simulink model "sampleModel2001_1_sub_sub_sub"  (R2023a)
settings: Solver=VariableStepAuto  StartTime=0.0  StopTime=10.0  RelTol=1e-3
libraries: hdlsllib x4, simulink x1
settings Model: Creator=user1  LastModifiedBy=user1
settings OptimizationCC: BlockReduction=off  ConditionallyExecuteInputs=off

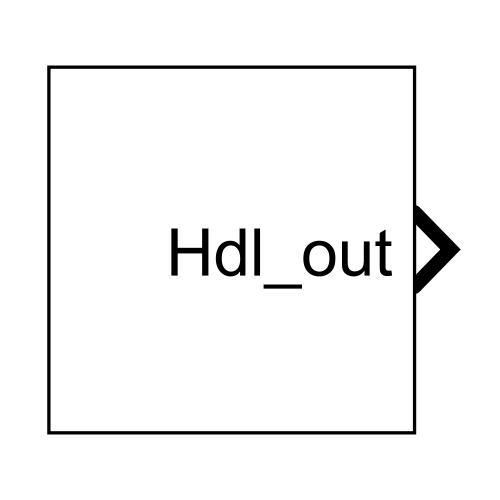
[thumbnail: Simulink's stored preview of the top-level diagram]
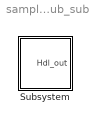
== system sampleModel2001_1_sub_sub_sub ==
  Subsystem : Subsystem

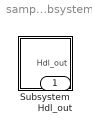
== system sampleModel2001_1_sub_sub_sub/Subsystem ==
  Subsystem : Subsystem
  Hdl_out : Outport  OutDataTypeStr=uint8

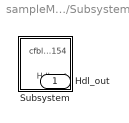
== system sampleModel2001_1_sub_sub_sub/Subsystem/Subsystem ==
  Subsystem : Subsystem
  Hdl_out : Outport  OutDataTypeStr=uint8

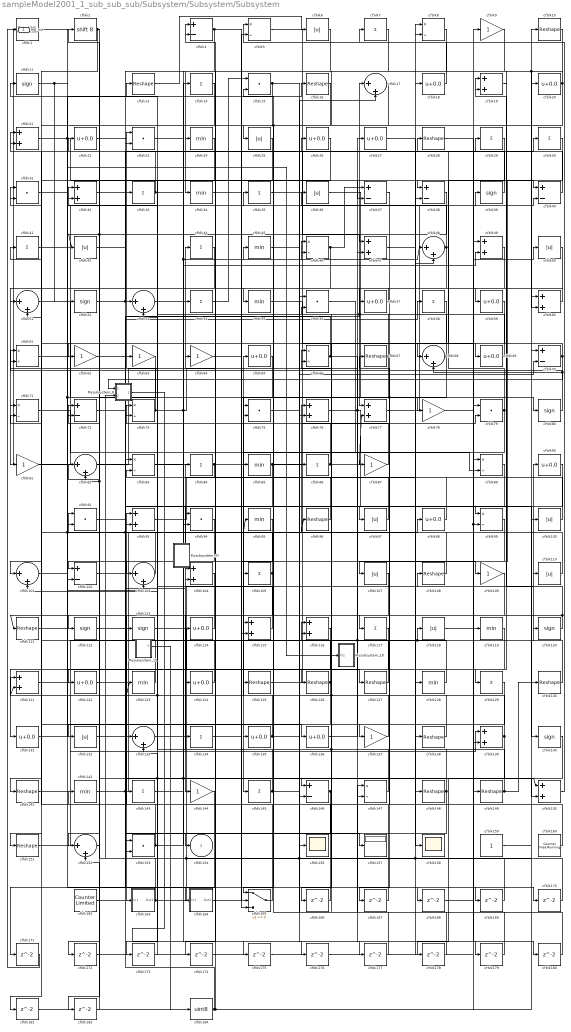
== system sampleModel2001_1_sub_sub_sub/Subsystem/Subsystem/Subsystem ==
  Mysubsystem_11 : Subsystem  TreatAsAtomicUnit=on  RTWFcnName=Mysubsystem_11
      settings: RTWFcnNameOpts=User specified  RTWFileNameOpts=Use function name
  Mysubsystem_19 : Subsystem  TreatAsAtomicUnit=on  RTWFcnName=Mysubsystem_19
      settings: RTWFcnNameOpts=User specified  RTWFileNameOpts=Use function name
  Mysubsystem_37 : Subsystem  TreatAsAtomicUnit=on  RTWFcnName=Mysubsystem_37
      settings: RTWFcnNameOpts=User specified  RTWFileNameOpts=Use function name
  Mysubsystem_8 : Subsystem  TreatAsAtomicUnit=on  RTWFcnName=Mysubsystem_8
      settings: RTWFcnNameOpts=User specified  RTWFileNameOpts=Use function name
  cfblk1 : hdlsllib/Logic and Bit Operations/Detect Fall Nonpositive  vinit=0  OutDataTypeStr=uint8
  cfblk{10,13,16,28,67,96,108,111,125..127,130,138,141,148..149,151} (17 alike) : Reshape
  cfblk{6,25,36,42,50,97,100,107,110,118,132} (11 alike) : Abs  OutDataTypeStr=uint8  SaturateOnIntegerOverflow=off
  cfblk{17,48,51,53,68,82,101,103,133,152} (10 alike) : Sum  Inputs=|++  OutDataTypeStr=uint8
  cfblk{4,37..38,40,70,72,102,146} (8 alike) : Sum  Inputs=+-  OutDataTypeStr=uint8
  cfblk{19,21,32,47,49,60,76..77,93,104,115..116,121,139,150} (15 alike) : Sum  OutDataTypeStr=uint8
  cfblk{7,14,29..30,33,35,41,44,54,58,84,86,105,117,129,134,143,145} (18 alike) : Sum  Inputs=+  OutDataTypeStr=uint8
  cfblk{9,62..64,78,81,87,109,137,144} (10 alike) : Gain  OutDataTypeStr=uint8
  cfblk{11,39,52,80,112..113,120,140} (8 alike) : Signum
  cfblk{18,20,22,26..27,57,59,65,69,90,98,114,122,124,131,135..136} (17 alike) : Bias  Bias=0.0  SaturateOnIntegerOverflow=off
  cfblk{24,34,45,55,85,95,119,123,128,142} (10 alike) : MinMax  OutDataTypeStr=uint8
  cfblk{5,8,46,61,66,71,73,83,89,99,147} (11 alike) : Product  Inputs=*/  OutDataTypeStr=uint8  RndMeth=Zero  SaturateOnIntegerOverflow=on
  cfblk{15,23,31,56,75,79,92,94,153} (9 alike) : DotProduct  OutDataTypeStr=uint8
  cfblk156 : Scope
  cfblk157 : Display
  cfblk158 : Scope
  cfblk159 : Constant  OutDataTypeStr=uint8  SampleTime=-1
  cfblk160 : hdlsllib/Sources/Counter Free-Running  NumBits=16  tsamp=-1
  cfblk162 : hdlsllib/Sources/Counter Limited  uplimit=7  tsamp=-1
  cfblk163 : Subsystem
      settings: LibrarySourceBlock=|
      | hdlsllib/Ports &
      | Subsystems/Subsystem
  cfblk164 : Subsystem
      settings: LibrarySourceBlock=|
      | hdlsllib/Ports &
      | Subsystems/Subsystem
  cfblk165 : Switch  OutDataTypeStr=uint8  SaturateOnIntegerOverflow=off  InputSameDT=off
  cfblk{166..182} (17 alike) : Delay  SampleTime=1
  cfblk184 : DataTypeConversion  OutDataTypeStr=uint8  SaturateOnIntegerOverflow=off  RndMeth=Floor
  cfblk2 : ArithShift  BitShiftNumber=8
  cfblk154 : Outport  OutDataTypeStr=uint8  VectorParamsAs1DForOutWhenUnconnected=off
  Hdl_out : Outport  Port=2  OutDataTypeStr=uint8
  wires:
  cfblk147/1 -> cfblk84/1
  cfblk125/1 -> cfblk29/1
  cfblk6/1 -> cfblk34/1
  cfblk57/1 -> cfblk55/1
  cfblk19/1 -> cfblk69/1
  cfblk54/1 -> cfblk15/1
  cfblk67/1 -> cfblk165/2, cfblk13/1, cfblk17/1
  cfblk81/1 -> cfblk35/1
  cfblk49/1 -> cfblk81/1
  cfblk30/1 -> cfblk107/1
  cfblk11/1 -> cfblk52/1, cfblk76/2, cfblk127/1
  cfblk50/1 -> cfblk77/1
  cfblk105/1 -> cfblk164/1(In1), cfblk41/1
  cfblk56/1 -> cfblk89/2
  cfblk142/1 -> cfblk115/1, cfblk98/1
  cfblk150/1 -> cfblk7/1
  cfblk44/1 -> cfblk71/1
  cfblk36/1 -> cfblk119/1
  cfblk62/1 -> cfblk23/1
  cfblk20/1 -> cfblk115/2, cfblk25/1
  cfblk114/1 -> cfblk112/1
  cfblk152/1 -> cfblk92/1
  cfblk115/1 -> cfblk32/1
  cfblk97/1 -> cfblk76/1
  cfblk46/1 -> cfblk37/1, cfblk51/1
  cfblk153/1 -> cfblk45/1, cfblk93/1
  cfblk27/1 -> cfblk158/1
  cfblk119/1 -> cfblk145/1
  cfblk130/1 -> cfblk90/1
  cfblk121/1 -> cfblk60/1
  cfblk35/1 -> cfblk38/1
  cfblk126/1 -> cfblk141/1, cfblk82/1
  cfblk113/1 -> cfblk126/1
  cfblk149/1 -> cfblk130/1, cfblk101/2, cfblk66/1
  cfblk34/1 -> cfblk109/1
  cfblk85/1 -> cfblk93/2, cfblk79/2
  cfblk77/1 -> cfblk9/1
  cfblk160/1 -> cfblk67/1
  cfblk128/1 -> cfblk118/1, cfblk63/1
  cfblk71/1 -> cfblk128/1
  cfblk4/1 -> cfblk37/2, cfblk24/1
  cfblk118/1 -> cfblk30/1
  cfblk21/1 -> cfblk148/1, Mysubsystem_19/1(In1)
  cfblk33/1 -> cfblk21/2, cfblk40/1
  cfblk163/1(Out1) -> cfblk110/1, cfblk146/2, cfblk8/2, cfblk10/1, Mysubsystem_8/2(In2)
  cfblk110/1 -> cfblk31/1
  cfblk89/1 -> cfblk104/1
  cfblk104/1 -> cfblk163/1(In1)
  cfblk66/1 -> cfblk150/2, cfblk53/1
  cfblk112/1 -> cfblk86/1
  cfblk109/1 -> cfblk137/1
  cfblk5/1 -> cfblk47/1
  cfblk10/1 -> cfblk60/2, cfblk129/1
  cfblk137/1 -> cfblk65/1
  cfblk84/1 -> cfblk83/2, cfblk154/1
  cfblk90/1 -> cfblk97/1
  cfblk73/1 -> cfblk31/2, cfblk169/1, cfblk47/2
  cfblk117/1 -> cfblk135/1
  cfblk136/1 -> cfblk108/1
  cfblk151/1 -> cfblk14/1
  cfblk42/1 -> cfblk146/1
  cfblk93/1 -> cfblk18/1
  cfblk47/1 -> cfblk138/1
  cfblk29/1 -> cfblk68/1
  cfblk18/1 -> cfblk5/1
  cfblk138/1 -> cfblk72/1
  cfblk92/1 -> cfblk57/1
  cfblk13/1 -> cfblk6/1
  cfblk82/1 -> cfblk44/1
  cfblk100/1 -> cfblk53/2
  cfblk40/1 -> cfblk19/1
  cfblk141/1 -> cfblk139/1
  cfblk116/1 -> cfblk131/1
  cfblk39/1 -> cfblk2/1
  cfblk41/1 -> cfblk20/1
  cfblk59/1 -> cfblk101/1
  cfblk159/1 -> cfblk70/1
  cfblk108/1 -> cfblk22/1
  cfblk111/1 -> cfblk16/1
  cfblk107/1 -> cfblk144/1
  cfblk61/1 -> cfblk134/1
  cfblk2/1 -> cfblk151/1, cfblk132/1
  cfblk25/1 -> cfblk124/1
  cfblk69/1 -> cfblk11/1
  cfblk51/1 -> cfblk78/1
  cfblk80/1 -> cfblk68/2, cfblk61/1
  cfblk120/1 -> cfblk19/2, cfblk111/1
  cfblk124/1 -> cfblk33/1
  cfblk65/1 -> cfblk125/1
  cfblk131/1 -> cfblk40/2, cfblk95/1
  cfblk103/1 -> cfblk71/2
  cfblk83/1 -> cfblk39/1, cfblk48/1
  cfblk53/1 -> cfblk54/1
  cfblk164/1(Out1) -> cfblk5/2
  cfblk148/1 -> cfblk153/2, cfblk73/1
  cfblk14/1 -> cfblk42/1, cfblk182/1, cfblk82/2
  cfblk16/1 -> cfblk85/1, cfblk51/2
  cfblk162/1 -> cfblk104/2
  cfblk146/1 -> cfblk153/1, cfblk116/1
  cfblk132/1 -> cfblk120/1
  cfblk76/1 -> cfblk179/1, cfblk140/1
  cfblk60/1 -> cfblk59/1
  cfblk95/1 -> cfblk103/1
  cfblk139/1 -> cfblk56/2, cfblk123/1, cfblk173/1, cfblk172/1
  cfblk134/1 -> cfblk46/1
  cfblk68/1 -> cfblk32/2, cfblk147/2, cfblk87/1
  cfblk15/1 -> cfblk165/3, cfblk80/1
  cfblk87/1 -> cfblk4/1
  cfblk63/1 -> cfblk102/1
  cfblk123/1 -> cfblk72/2
  cfblk78/1 -> cfblk50/1
  cfblk24/1 -> cfblk143/1
  cfblk70/1 -> cfblk62/1, Mysubsystem_8/1(In1)
  cfblk64/1 -> cfblk46/2
  cfblk102/1 -> cfblk58/1, cfblk96/1
  cfblk135/1 -> cfblk17/2, cfblk121/1
  cfblk94/1 -> cfblk102/2
  cfblk1/1 -> cfblk133/1
  cfblk52/1 -> cfblk28/1, cfblk136/1
  cfblk38/1 -> cfblk152/1
  cfblk8/1 -> cfblk23/2
  cfblk98/1 -> cfblk75/1
  cfblk9/1 -> cfblk94/1
  cfblk32/1 -> cfblk157/1
  cfblk79/1 -> cfblk105/1, cfblk26/1
  cfblk127/1 -> cfblk21/1
  cfblk99/1 -> cfblk117/1
  cfblk7/1 -> cfblk94/2
  cfblk96/1 -> cfblk75/2
  cfblk165/1 -> cfblk142/1
  cfblk75/1 -> cfblk156/1
  cfblk86/1 -> Hdl_out/1, cfblk73/2, cfblk77/2
  cfblk55/1 -> cfblk99/2, cfblk149/1
  cfblk145/1 -> cfblk70/2, cfblk121/2, cfblk113/1
  cfblk17/1 -> cfblk122/1
  cfblk48/1 -> cfblk165/1, cfblk36/1
  cfblk133/1 -> cfblk49/2
  cfblk143/1 -> cfblk150/1, cfblk114/1
  cfblk101/1 -> cfblk103/2
  cfblk22/1 -> cfblk99/1
  cfblk122/1 -> cfblk8/1, cfblk27/1
  cfblk58/1 -> cfblk166/1
  cfblk166/1 -> cfblk61/2
  cfblk37/1 -> cfblk167/1
  cfblk167/1 -> cfblk66/2
  cfblk31/1 -> cfblk168/1
  cfblk168/1 -> cfblk49/1
  cfblk169/1 -> cfblk4/2
  cfblk72/1 -> cfblk170/1
  cfblk170/1 -> cfblk92/2
  cfblk144/1 -> cfblk171/1
  cfblk171/1 -> cfblk1/1
  cfblk172/1 -> cfblk38/2
  cfblk173/1 -> cfblk133/2
  cfblk129/1 -> cfblk174/1
  cfblk174/1 -> cfblk48/2
  cfblk23/1 -> cfblk175/1
  cfblk175/1 -> cfblk89/1
  cfblk176/1 -> cfblk139/2
  cfblk45/1 -> cfblk177/1
  cfblk177/1 -> cfblk116/2
  cfblk140/1 -> cfblk178/1
  cfblk178/1 -> cfblk15/2
  cfblk179/1 -> cfblk56/1
  cfblk28/1 -> cfblk180/1
  cfblk180/1 -> cfblk147/1
  cfblk26/1 -> cfblk181/1
  cfblk181/1 -> cfblk79/1
  cfblk182/1 -> cfblk152/2
  cfblk184/1 -> cfblk83/1, cfblk64/1, cfblk100/1
  Mysubsystem_8/1(Out1) -> cfblk176/1
  Mysubsystem_11/1(Y) -> cfblk184/1

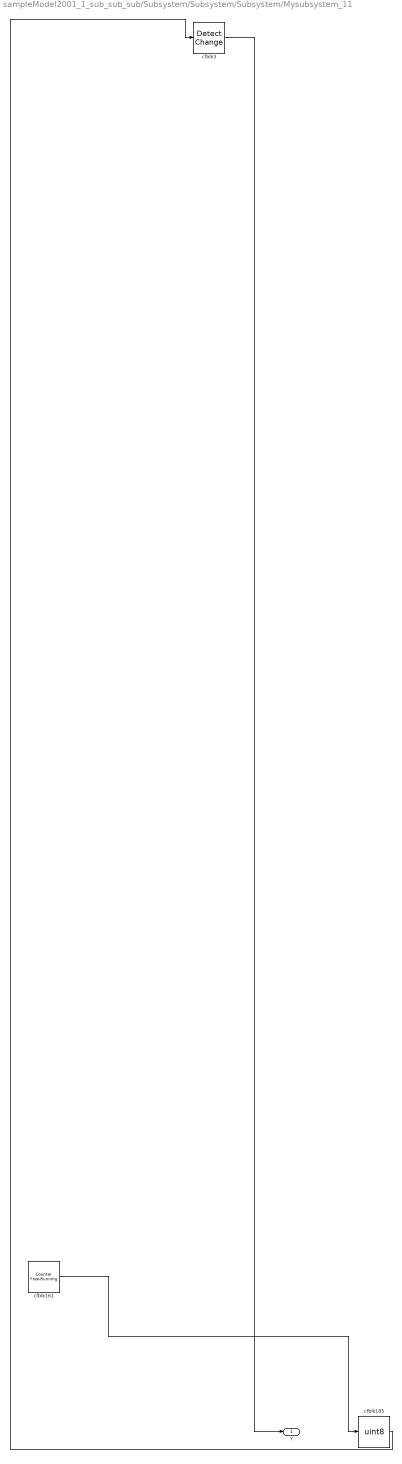
== system sampleModel2001_1_sub_sub_sub/Subsystem/Subsystem/Subsystem/Mysubsystem_11 ==
  cfblk161 : hdlsllib/Sources/Counter Free-Running  NumBits=16  tsamp=-1
  cfblk185 : DataTypeConversion  OutDataTypeStr=uint8  SaturateOnIntegerOverflow=off  RndMeth=Floor
  cfblk3 : simulink/Logic and Bit Operations/Detect Change  vinit=0  OutDataTypeStr=boolean
      settings: LibrarySourceBlock=|
      | hdlsllib/Logic and Bit
      | Operations/Detect
      | Change
  Y : Outport
  wires:
  cfblk3/1 -> Y/1
  cfblk185/1 -> cfblk3/1
  cfblk161/1 -> cfblk185/1

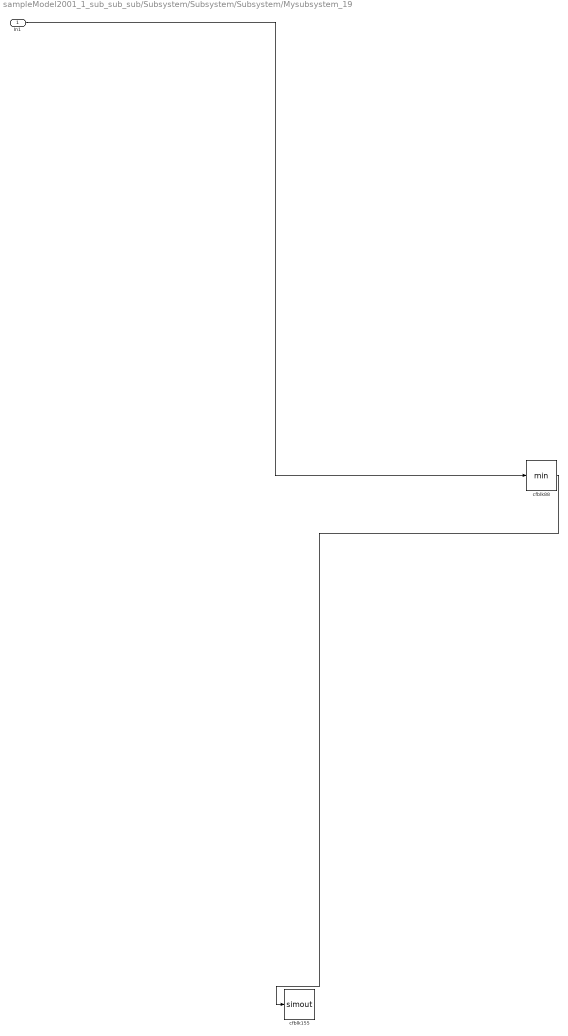
== system sampleModel2001_1_sub_sub_sub/Subsystem/Subsystem/Subsystem/Mysubsystem_19 ==
  In1 : Inport
  cfblk155 : ToWorkspace  VariableName=simout  SaveFormat=Timeseries  SampleTime=-1
  cfblk88 : MinMax
  wires:
  In1/1 -> cfblk88/1
  cfblk88/1 -> cfblk155/1

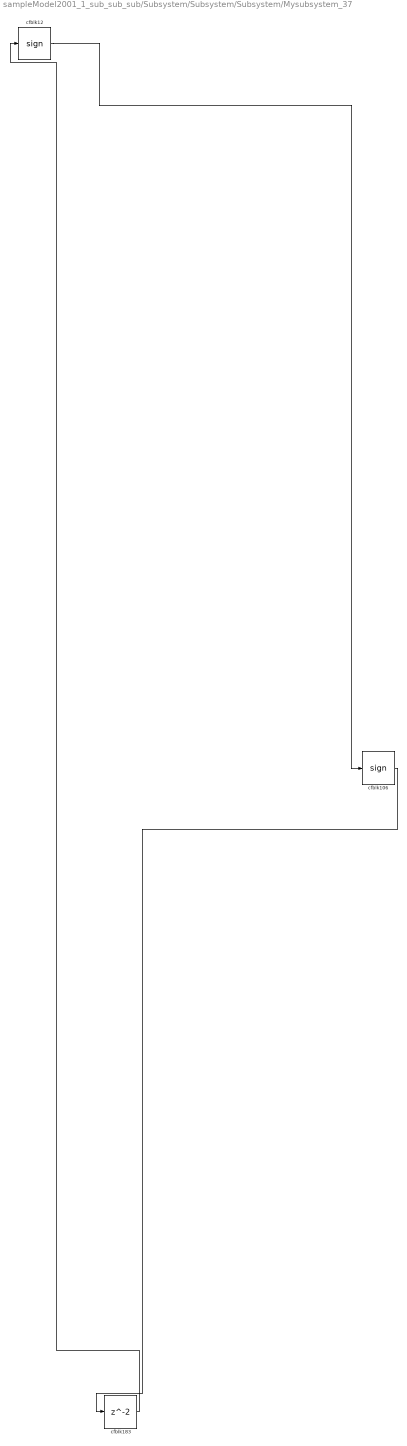
== system sampleModel2001_1_sub_sub_sub/Subsystem/Subsystem/Subsystem/Mysubsystem_37 ==
  cfblk106 : Signum
  cfblk12 : Signum
  cfblk183 : Delay  SampleTime=1
  wires:
  cfblk12/1 -> cfblk106/1
  cfblk183/1 -> cfblk12/1
  cfblk106/1 -> cfblk183/1

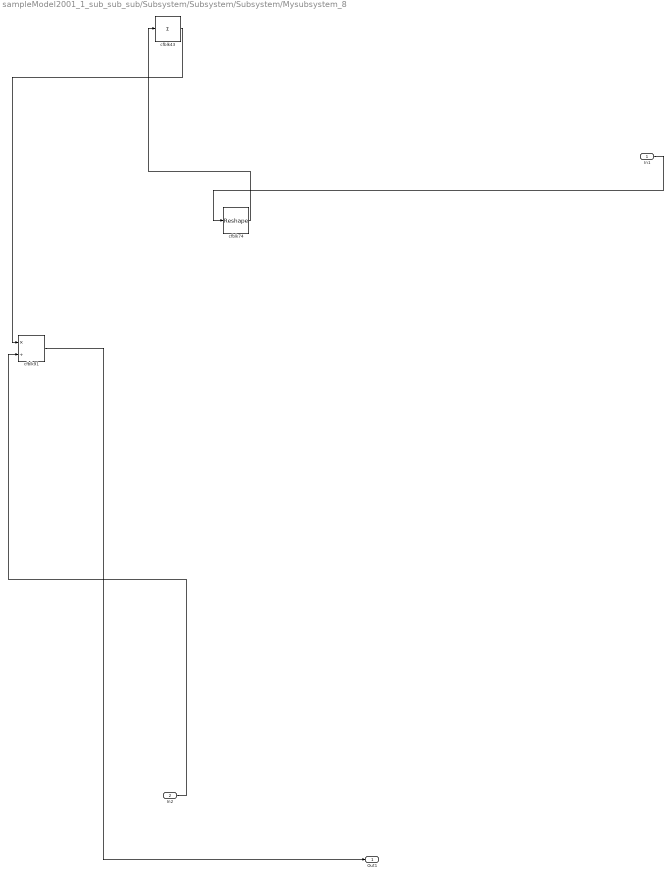
== system sampleModel2001_1_sub_sub_sub/Subsystem/Subsystem/Subsystem/Mysubsystem_8 ==
  In1 : Inport
  In2 : Inport  Port=2
  cfblk43 : Sum  Inputs=+
  cfblk74 : Reshape
  cfblk91 : Product  Inputs=*/  RndMeth=Zero  SaturateOnIntegerOverflow=on
  Out1 : Outport
  wires:
  cfblk74/1 -> cfblk43/1
  In1/1 -> cfblk74/1
  cfblk91/1 -> Out1/1
  In2/1 -> cfblk91/2
  cfblk43/1 -> cfblk91/1

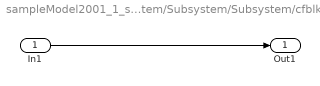
== system sampleModel2001_1_sub_sub_sub/Subsystem/Subsystem/Subsystem/cfblk163 ==
  In1 : Inport
  Out1 : Outport
  wires:
  In1/1 -> Out1/1

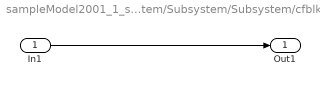
== system sampleModel2001_1_sub_sub_sub/Subsystem/Subsystem/Subsystem/cfblk164 ==
  In1 : Inport
  Out1 : Outport
  wires:
  In1/1 -> Out1/1
